simulink model "MTHNYI011_Kitti_Model_LAB2"  (R2023a)
settings: Solver=VariableStepAuto  StartTime=0.0  StopTime=270  RelTol=1e-3
libraries: spspowerguiLib x1
settings Model: LastModifiedBy=Nyiko
settings RTWCC: GPUComputeCapability=5.0
settings ConfigComp: CovBoundaryAbsTol=1.0e-5

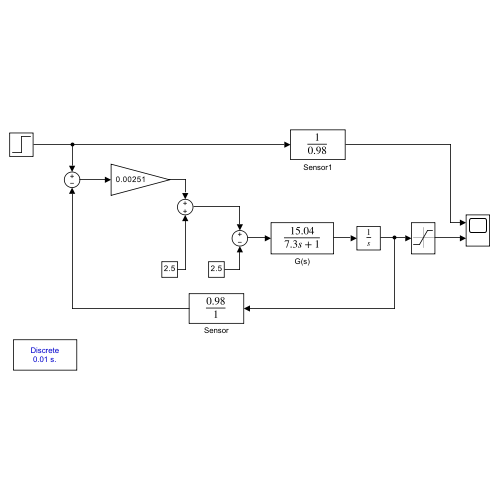
[thumbnail: Simulink's stored preview of the top-level diagram]
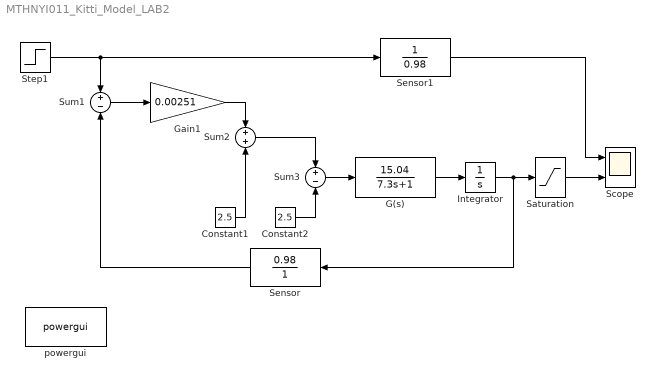
== system MTHNYI011_Kitti_Model_LAB2 ==
  Constant1 : Constant  Value=2.5
  Constant2 : Constant  Value=2.5
  G(s) : TransferFcn  Numerator=[15.04]  Denominator=[7.3 1]
  Gain1 : Gain  Gain=0.00251
  Integrator : Integrator
  Saturation : Saturate  UpperLimit=5  LowerLimit=0
  Scope : Scope  NumInputPorts=2
  Sensor : TransferFcn  Numerator=[0.98]  Denominator=[1]
  Sensor1 : TransferFcn  Denominator=[0.98]
  Step1 : Step  Time=0  After=2.5  SampleTime=0
  Sum1 : Sum  Inputs=+-
  Sum2 : Sum
  Sum3 : Sum  Inputs=+-
  powergui : spspowerguiLib/powergui  Priority=1  SimulationMode=Discrete  SampleTime=10e-3  frequency=60  Iterations=50  frequencyindice=60  Pbase=100e6  ErrMax=1e-4  UnitsV=kV  UnitsW=MW  buscounter=0  FunctionMessages=off  echomessages=off  EnableUseOfTLC=off  CurrentSourceSwitches=off  DisableSnubberDevices=off  DisableRonSwitches=off  DisableVfSwitches=off  DisplayEquations=off  AutomaticDiscreteSolvers=off  SolverType=Tustin/Backward Euler (TBE)  Interpol=off  ExternalGateDelay=off  methode=off  Ts=100  x0status=blocks  SPID=on  SwTol=0  HookPort=off  NonlinearTolerance=1e-4  nMaxIteration=100  ContinueOnMaxIteration=off  RestoreLinks=warning  ResistiveCurrentMeasurement=off  Frange=[0:2:500]  Ylog=off  Xlog=on  ShowGrid=off  save=off  variable=ZData  structure=0  ZoomFFT=off  StartTime=0.0  cycles=1  DisplayStyle=1  fundamental=60  FreqAxis=off  MaxFrequency=1000  frequencyindicesteady=1  RmsSteady=1  display=off
  wires:
  Gain1/1 -> Sum2/1
  Constant1/1 -> Sum2/2
  Sum2/1 -> Sum3/1
  Constant2/1 -> Sum3/2
  Sum3/1 -> G(s)/1
  G(s)/1 -> Integrator/1
  Step1/1 -> Sum1/1, Sensor1/1
  Integrator/1 -> Sensor/1, Saturation/1
  Sensor/1 -> Sum1/2
  Sum1/1 -> Gain1/1
  Saturation/1 -> Scope/2
  Sensor1/1 -> Scope/1
